simulink model "tmp3"  (R2017a)
settings: Solver=VariableStepAuto  StartTime=0.0  StopTime=simTime  RelTol=1e-3
values from neighbouring files (symbols this model uses):
  dt = 0.1    [exmM_IM.m]
settings Model: Creator=lzr96  LastModifiedBy=lzr96

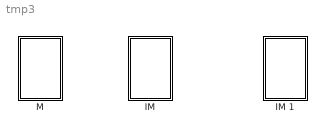
== system tmp3 ==
  "IM " : Subsystem
      mask Display: disp('IM序列')
  IM 1 : Subsystem
      mask Display: disp('IM序列')
  M : Subsystem
      mask Display: disp('M序列')

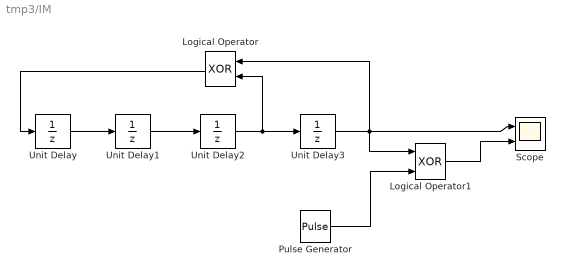
== system tmp3/IM  ==
  Logical Operator : Logic  Operator=XOR  AllPortsSameDT=off  OutDataTypeStr=boolean
  Logical Operator1 : Logic  Operator=XOR  AllPortsSameDT=off  OutDataTypeStr=boolean
  Pulse Generator : DiscretePulseGenerator  PulseType=Time based  Period=dt*2  PulseWidth=50
  Scope : Scope  NumInputPorts=2
  Unit Delay : UnitDelay  InitialCondition=1  SampleTime=-1
  Unit Delay1 : UnitDelay  SampleTime=-1
  Unit Delay2 : UnitDelay  SampleTime=-1
  Unit Delay3 : UnitDelay  SampleTime=-1
  wires:
  Unit Delay/1 -> Unit Delay1/1
  Unit Delay1/1 -> Unit Delay2/1
  Pulse Generator/1 -> Logical Operator1/2
  Unit Delay2/1 -> Logical Operator/2, Unit Delay3/1
  Logical Operator/1 -> Unit Delay/1
  Logical Operator1/1 -> Scope/2
  Unit Delay3/1 -> Scope/1, Logical Operator/1, Logical Operator1/1

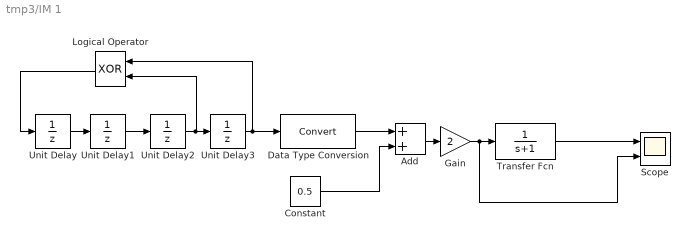
== system tmp3/IM 1 ==
  Add : Sum
  Constant : Constant  Value=0.5
  Data Type Conversion : DataTypeConversion
  Gain : Gain  Gain=2
  Logical Operator : Logic  Operator=XOR  AllPortsSameDT=off  OutDataTypeStr=boolean
  Scope : Scope  NumInputPorts=2
  Transfer Fcn : TransferFcn  Denominator=[1 1]
  Unit Delay : UnitDelay  InitialCondition=1  SampleTime=-1
  Unit Delay1 : UnitDelay  SampleTime=-1
  Unit Delay2 : UnitDelay  SampleTime=-1
  Unit Delay3 : UnitDelay  SampleTime=-1
  wires:
  Unit Delay3/1 -> Data Type Conversion/1, Logical Operator/1
  Logical Operator/1 -> Unit Delay/1
  Unit Delay2/1 -> Logical Operator/2, Unit Delay3/1
  Unit Delay1/1 -> Unit Delay2/1
  Unit Delay/1 -> Unit Delay1/1
  Data Type Conversion/1 -> Add/1
  Constant/1 -> Add/2
  Add/1 -> Gain/1
  Gain/1 -> Scope/2, Transfer Fcn/1
  Transfer Fcn/1 -> Scope/1

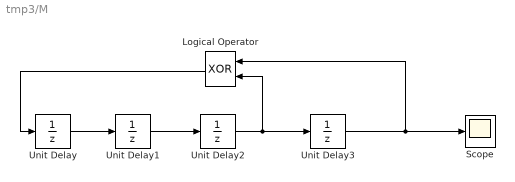
== system tmp3/M ==
  Logical Operator : Logic  Operator=XOR  AllPortsSameDT=off  OutDataTypeStr=boolean
  Scope : Scope
  Unit Delay : UnitDelay  InitialCondition=1  SampleTime=-1
  Unit Delay1 : UnitDelay  SampleTime=-1
  Unit Delay2 : UnitDelay  SampleTime=-1
  Unit Delay3 : UnitDelay  SampleTime=-1
  wires:
  Unit Delay/1 -> Unit Delay1/1
  Unit Delay3/1 -> Scope/1, Logical Operator/1
  Unit Delay1/1 -> Unit Delay2/1
  Logical Operator/1 -> Unit Delay/1
  Unit Delay2/1 -> Logical Operator/2, Unit Delay3/1
